simulink model "planta_segway_v1"  (R2023b)
settings: Solver=ode15s  StartTime=0.0  StopTime=Tfin  MaxStep=2e-3  RelTol=1e-5  AbsTol=1e-7
values from neighbouring files (symbols this model uses):
  meas0 = repmat(meas0, [1 1 max(E.n_delay, 1)])    [cargar_workspace_v1.m]    (also in medida_inicial_v1.m = sensores_sl(X0, y0, zeros(3,1), pv))
  pv = empaquetar_v1(P, C)    [cargar_workspace_v1.m]    (also in empaquetar_v1.m = zeros(124,1); simular_ode_v1.m)
  Ts = pv(40)    [control_v1.m]    (also in simular_ode_v1.m = P.sens.Ts; simular_slx_v1.m = P.sens.Ts)
  X0 = zeros(16,1); X0(3) = P.din.l0    [escenarios_v1.m]
undefined symbols (not defined in the file or in its folder): n_delay, semilla
settings Model: Creator=calde  LastModifiedBy=calde

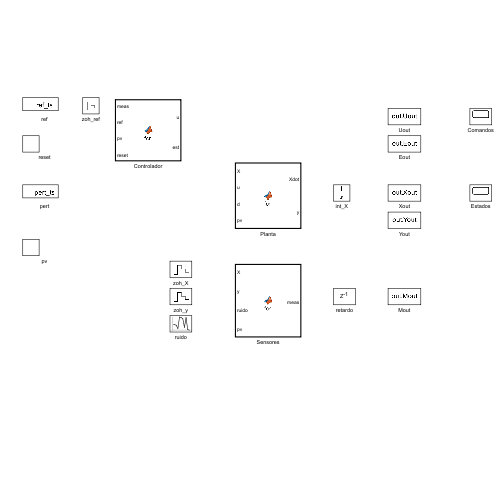
[thumbnail: Simulink's stored preview of the top-level diagram]
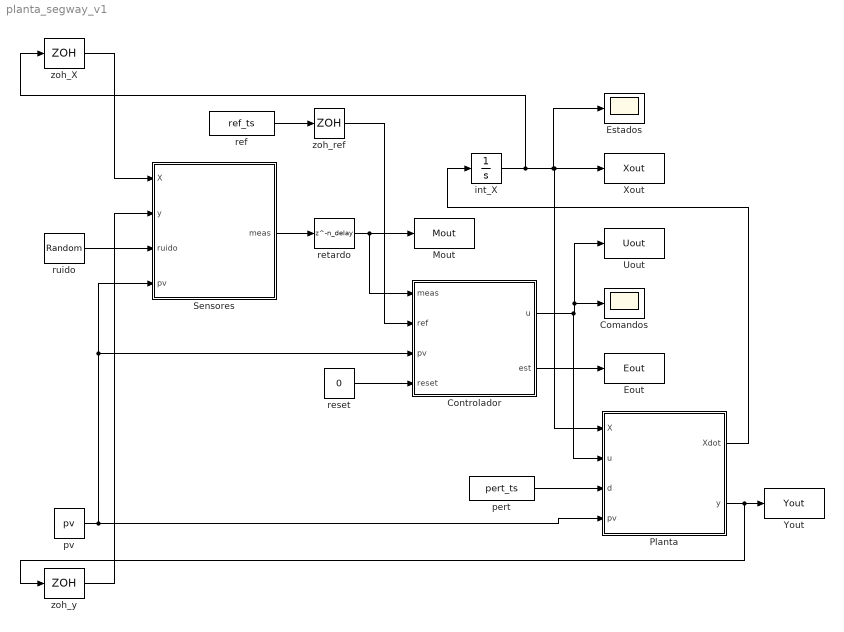
== system planta_segway_v1 ==
  Comandos : Scope
  Controlador : MATLAB Function  TreatAsAtomicUnit=on
  Eout : ToWorkspace  VariableName=Eout  SaveFormat=Structure With Time  SampleTime=-1
  Estados : Scope
  Mout : ToWorkspace  VariableName=Mout  SaveFormat=Structure With Time  SampleTime=-1
  Planta : MATLAB Function  TreatAsAtomicUnit=on
  Sensores : MATLAB Function  TreatAsAtomicUnit=on
  Uout : ToWorkspace  VariableName=Uout  SaveFormat=Structure With Time  SampleTime=-1
  Xout : ToWorkspace  VariableName=Xout  SaveFormat=Structure With Time  SampleTime=-1
  Yout : ToWorkspace  VariableName=Yout  SaveFormat=Structure With Time  SampleTime=-1
  int_X : Integrator  InitialCondition=X0
  pert : FromWorkspace  VariableName=pert_ts  Interpolate=off  OutputAfterFinalValue=Holding final value
  pv : Constant  Value=pv
  ref : FromWorkspace  VariableName=ref_ts  SampleTime=Ts  Interpolate=off  OutputAfterFinalValue=Holding final value
  reset : Constant  Value=0  SampleTime=Ts
  retardo : Delay  DelayLength=n_delay  InitialCondition=meas0  SampleTime=Ts
  ruido : RandomNumber  Seed=semilla+[0 1 2]  SampleTime=Ts
  zoh_X : ZeroOrderHold  SampleTime=Ts
  zoh_ref : ZeroOrderHold  SampleTime=Ts
  zoh_y : ZeroOrderHold  SampleTime=Ts
  wires:
  zoh_y/1 -> Sensores/2(y)
  zoh_X/1 -> Sensores/1(X)
  ruido/1 -> Sensores/3(ruido)
  ref/1 -> zoh_ref/1
  pv/1 -> Controlador/3(pv), Sensores/4(pv), Planta/4(pv)
  Sensores/1(meas) -> retardo/1
  zoh_ref/1 -> Controlador/2(ref)
  int_X/1 -> Planta/1(X), Xout/1, Estados/1, zoh_X/1
  retardo/1 -> Controlador/1(meas), Mout/1
  reset/1 -> Controlador/4(reset)
  Controlador/1(u) -> Uout/1, Comandos/1, Planta/2(u)
  Controlador/2(est) -> Eout/1
  pert/1 -> Planta/3(d)
  Planta/1(Xdot) -> int_X/1
  Planta/2(y) -> zoh_y/1, Yout/1

== matlab function planta_segway_v1/Planta ==
  data: X input; Xdot output; u input; y output; d input; pv input
function [Xdot, y] = fcn(X, u, d, pv)
%#codegen
[Xdot, y] = planta_sl(X, u, d, pv);

== matlab function planta_segway_v1/Controlador ==
  data: meas input; u output; ref input; pv input; reset input; est output
function [u, est] = fcn(meas, ref, pv, reset)
%#codegen
[u, est] = control_v1(meas, ref, pv, reset);

== matlab function planta_segway_v1/Sensores ==
  data: X input; meas output; y input; ruido input; pv input
function meas = fcn(X, y, ruido, pv)
%#codegen
meas = sensores_sl(X, y, ruido, pv);
